simulink model "ESTS_VSLARE_test"  (R2024b)
settings: Solver=VariableStepAuto  StartTime=0.0  StopTime=10.0  RelTol=1e-3
libraries: ESTS_VSLARE x1
settings Model: Creator=blatak  LastModifiedBy=blatak

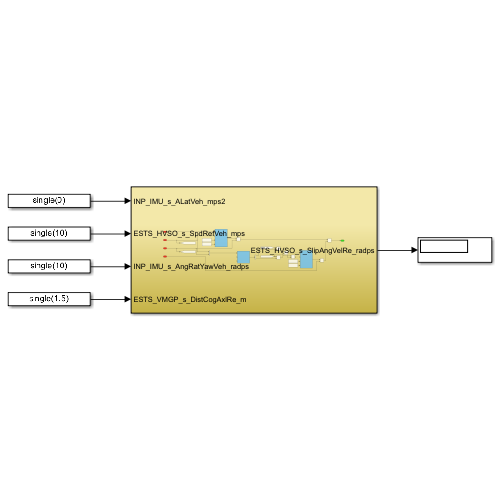
[thumbnail: Simulink's stored preview of the top-level diagram]
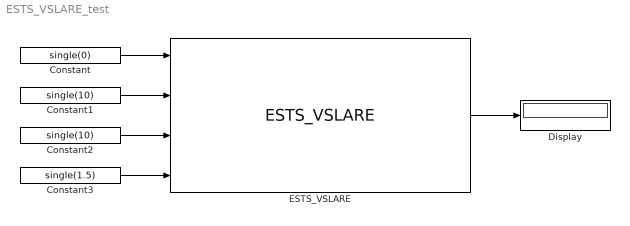
== system ESTS_VSLARE_test ==
  Constant : Constant  Value=single(0)
  Constant1 : Constant  Value=single(10)
  Constant2 : Constant  Value=single(10)
  Constant3 : Constant  Value=single(1.5)
  Display : Display
  ESTS_VSLARE : ESTS_VSLARE/ESTS_VSLARE  SystemSampleTime=-1  VariantActivationTime=update diagram  AllowFlexibleInterface=on  Latency=0  AutoFrameSizeCalculation=off
  wires:
  Constant/1 -> ESTS_VSLARE/1
  Constant1/1 -> ESTS_VSLARE/2
  Constant2/1 -> ESTS_VSLARE/3
  Constant3/1 -> ESTS_VSLARE/4
  ESTS_VSLARE/1 -> Display/1
